simulink model "SC617_Final"  (R2025a)
settings: Solver=ode15s  StartTime=0.0  StopTime=30  MaxStep=0.05  RelTol=1e-2  AbsTol=1e-2
undefined symbols (not defined in the file): magnitude
settings Model: Creator=aayushshah  LastModifiedBy=aayushshah

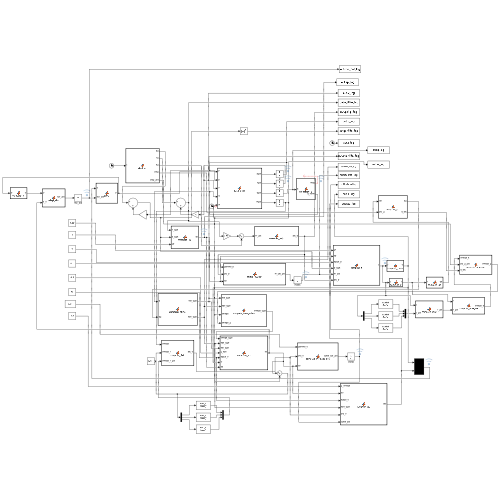
[thumbnail: Simulink's stored preview of the top-level diagram]
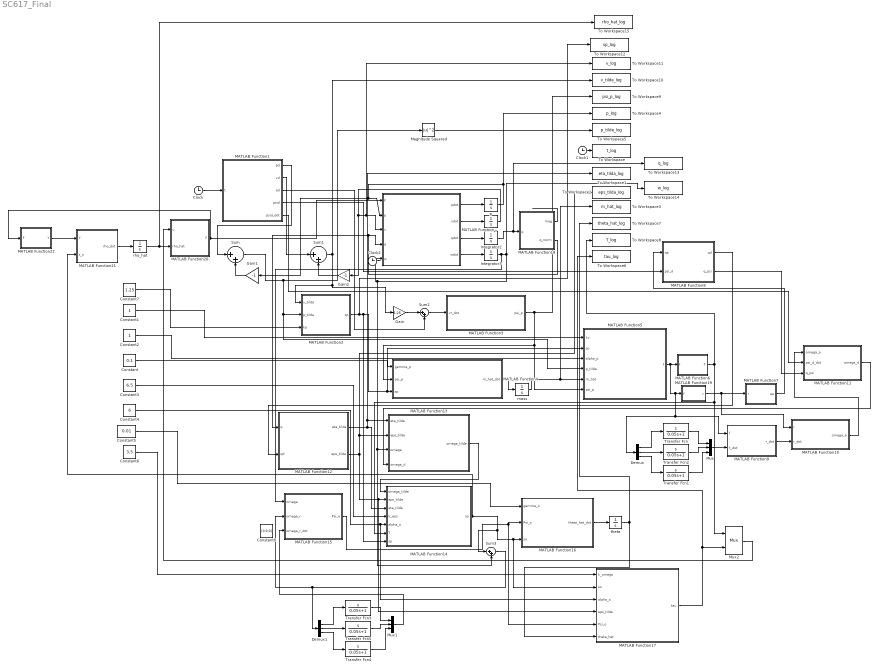
== system SC617_Final ==
  Clock : Clock
  Clock1 : Clock
  Clock2 : Clock
  Constant : Constant  Value=0.1
  Constant1 : Constant
  Constant2 : Constant
  Constant3 : Constant  Value=6.5
  Constant4 : Constant  Value=6
  Constant5 : Constant  Value=0.01
  Constant6 : Constant  Value=3.5
  Constant7 : Constant  Value=1.25
  Constant8 : Constant  Value=[0;0;0]
  Demux : Demux  Outputs=3
  Demux1 : Demux  Outputs=3
  Gain : Gain  Gain=1.25
  Gain1 : Gain  Gain=-1
  Gain2 : Gain  Gain=-1
  Integrator2 : Integrator  InitialCondition=[1; 0; 0; 0]
  Integrator3 : Integrator  InitialCondition=[0; 0; 0]
  MATLAB Function : MATLAB Function  TreatAsAtomicUnit=on
  MATLAB Function1 : MATLAB Function  TreatAsAtomicUnit=on
  MATLAB Function10 : MATLAB Function  TreatAsAtomicUnit=on
  MATLAB Function11 : MATLAB Function  TreatAsAtomicUnit=on
  MATLAB Function12 : MATLAB Function  TreatAsAtomicUnit=on
  MATLAB Function13 : MATLAB Function  TreatAsAtomicUnit=on
  MATLAB Function14 : MATLAB Function  TreatAsAtomicUnit=on
  MATLAB Function15 : MATLAB Function  TreatAsAtomicUnit=on
  MATLAB Function16 : MATLAB Function  TreatAsAtomicUnit=on
  MATLAB Function17 : MATLAB Function  TreatAsAtomicUnit=on
  MATLAB Function18 : MATLAB Function  TreatAsAtomicUnit=on
  MATLAB Function19 : MATLAB Function  TreatAsAtomicUnit=on
  MATLAB Function2 : MATLAB Function  TreatAsAtomicUnit=on
  MATLAB Function20 : MATLAB Function  TreatAsAtomicUnit=on
  MATLAB Function21 : MATLAB Function  TreatAsAtomicUnit=on
  MATLAB Function22 : MATLAB Function  TreatAsAtomicUnit=on
  MATLAB Function3 : MATLAB Function  TreatAsAtomicUnit=on
  MATLAB Function4 : MATLAB Function  TreatAsAtomicUnit=on
  MATLAB Function5 : MATLAB Function  TreatAsAtomicUnit=on
  MATLAB Function6 : MATLAB Function  TreatAsAtomicUnit=on
  MATLAB Function7 : MATLAB Function  TreatAsAtomicUnit=on
  MATLAB Function8 : MATLAB Function  TreatAsAtomicUnit=on
  MATLAB Function9 : MATLAB Function  TreatAsAtomicUnit=on
  Magnitude Squared : Math  Operator=magnitude^2
  Mux : Mux  Inputs=3
  Mux1 : Mux  Inputs=3
  Mux2 : Mux  Inputs=2
  Sum{,1..3} (4 alike) : Sum  Inputs=|++
  To Workspace : ToWorkspace  VariableName=t_log  SampleTime=-1
      settings: Decimation=50  Save2DSignal=2-D array (concatenate along first dimension)
  To Workspace1 : ToWorkspace  VariableName=eta_tilda_log  SampleTime=-1
      settings: Decimation=50  Save2DSignal=2-D array (concatenate along first dimension)
  To Workspace10 : ToWorkspace  VariableName=v_tilde_log  SampleTime=-1
      settings: Decimation=50  Save2DSignal=2-D array (concatenate along first dimension)
  To Workspace11 : ToWorkspace  VariableName=v_log  SampleTime=-1
      settings: Decimation=50  Save2DSignal=2-D array (concatenate along first dimension)
  To Workspace12 : ToWorkspace  VariableName=sp_log  SampleTime=-1
  To Workspace13 : ToWorkspace  VariableName=q_log  SampleTime=-1
      settings: Decimation=50  Save2DSignal=2-D array (concatenate along first dimension)
  To Workspace14 : ToWorkspace  VariableName=w_log  SampleTime=-1
      settings: Decimation=50  Save2DSignal=2-D array (concatenate along first dimension)
  To Workspace15 : ToWorkspace  VariableName=rho_hat_log  SampleTime=-1
  To Workspace2 : ToWorkspace  VariableName=eps_tilda_log  SampleTime=-1
      settings: Decimation=50  Save2DSignal=2-D array (concatenate along first dimension)
  To Workspace3 : ToWorkspace  VariableName=m_hat_log  SampleTime=-1
      settings: Decimation=50  Save2DSignal=2-D array (concatenate along first dimension)
  To Workspace4 : ToWorkspace  VariableName=p_log  SampleTime=-1
      settings: Decimation=50  Save2DSignal=2-D array (concatenate along first dimension)
  To Workspace5 : ToWorkspace  VariableName=p_tilde_log  SampleTime=-1
      settings: Decimation=50  Save2DSignal=2-D array (concatenate along first dimension)
  To Workspace6 : ToWorkspace  VariableName=tau_log  SampleTime=-1
      settings: Decimation=50  Save2DSignal=2-D array (concatenate along first dimension)
  To Workspace7 : ToWorkspace  VariableName=theta_hat_log  SampleTime=-1
      settings: Decimation=50  Save2DSignal=2-D array (concatenate along first dimension)
  To Workspace8 : ToWorkspace  VariableName=T_log  SampleTime=-1
      settings: Decimation=50  Save2DSignal=2-D array (concatenate along first dimension)
  To Workspace9 : ToWorkspace  VariableName=psi_p_log  SampleTime=-1
      settings: Decimation=50  Save2DSignal=2-D array (concatenate along first dimension)
  Transfer Fcn{,1..5} (6 alike) : TransferFcn  Numerator=[1 0]  Denominator=[0.05 1]
  mass : Integrator  InitialCondition=0.8
  p : Integrator  InitialCondition=[4.0; 0.5; 1.0]
  rho_hat : Integrator  InitialCondition=[0.18; 0.009]
  theta : Integrator  InitialCondition=[0.05; 0.05; 0.01]
  v : Integrator  InitialCondition=[0; 0; 0]
  wires:
  MATLAB Function/1(pdot) -> p/1
  MATLAB Function/2(vdot) -> v/1
  MATLAB Function/3(qdot) -> Integrator2/1
  MATLAB Function/4(wdot) -> Integrator3/1
  p/1 -> To Workspace4/1, MATLAB Function/2(p), Gain1/1
  v/1 -> Gain2/1, To Workspace11/1, MATLAB Function/3(v)
  Integrator3/1 -> MATLAB Function15/1(omega), To Workspace14/1, MATLAB Function13/3(omega), Sum3/2, MATLAB Function/5(w)
  Integrator2/1 -> To Workspace13/1, MATLAB Function18/1(q)
  MATLAB Function18/2(q_norm) -> MATLAB Function/4(q), MATLAB Function12/1(q)
  Clock/1 -> MATLAB Function1/1(t)
  MATLAB Function1/1(pd) -> Sum/1
  MATLAB Function1/2(vd) -> Sum1/1
  Sum/1 -> Magnitude Squared/1, MATLAB Function5/4(p_tilda), MATLAB Function2/2(p_tilda)
  Sum1/1 -> MATLAB Function2/1(v_tilda), Gain/1, To Workspace10/1
  Gain/1 -> Sum2/1
  MATLAB Function1/3(ad) -> Sum2/2
  Sum2/1 -> MATLAB Function3/1(vr_dot)
  MATLAB Function2/1(sp) -> To Workspace12/1, MATLAB Function14/7(sp), MATLAB Function5/2(sp), MATLAB Function4/3(sp)
  MATLAB Function3/1(psi_p) -> To Workspace9/1, MATLAB Function5/6(psi_p), MATLAB Function4/2(psi_p)
  Constant/1 -> MATLAB Function4/1(gamma_p)
  Constant1/1 -> MATLAB Function5/1(kv)
  Constant2/1 -> MATLAB Function5/3(alpha_p)
  MATLAB Function5/1(f) -> Demux/1, MATLAB Function9/1(f), MATLAB Function19/1(f), MATLAB Function6/1(f)
  MATLAB Function19/1(r) -> MATLAB Function10/1(r), MATLAB Function7/1(r)
  MATLAB Function7/1(qa) -> MATLAB Function8/1(qa)
  MATLAB Function1/4(psid) -> MATLAB Function8/2(psi_d)
  Demux/1 -> Transfer Fcn/1
  Demux/2 -> Transfer Fcn2/1
  Demux/3 -> Transfer Fcn1/1
  Transfer Fcn/1 -> Mux/1
  Transfer Fcn2/1 -> Mux/2
  Transfer Fcn1/1 -> Mux/3
  MATLAB Function9/1(r_dot) -> MATLAB Function10/2(r_dot)
  MATLAB Function10/1(omega_a) -> MATLAB Function11/1(omega_a)
  MATLAB Function8/2(q_psi) -> MATLAB Function11/3(q_psi)
  MATLAB Function1/5(psid_dot) -> MATLAB Function11/2(psi_d_dot)
  MATLAB Function8/1(qd) -> MATLAB Function12/2(qd)
  MATLAB Function12/1(eta_tilda) -> To Workspace1/1, MATLAB Function13/1(eta_tilde), MATLAB Function14/3(eta_tilde)
  MATLAB Function12/2(eps_tilda) -> MATLAB Function13/2(eps_tilde), To Workspace2/1, MATLAB Function14/2(eps_tilde), MATLAB Function17/4(eps_tilde)
  MATLAB Function11/1(omega_d) -> MATLAB Function13/4(omega_d)
  MATLAB Function13/1(omega_tilde) -> MATLAB Function14/1(omega_tilde)
  MATLAB Function6/1(T) -> To Workspace8/1, Mux2/1, MATLAB Function14/6(T)
  Constant3/1 -> MATLAB Function14/4(k_eps)
  Constant4/1 -> MATLAB Function17/3(alpha_o), MATLAB Function14/5(alpha_o)
  MATLAB Function14/1(so) -> MATLAB Function21/2(s_o), MATLAB Function16/3(so), MATLAB Function17/2(so), Sum3/1
  MATLAB Function15/1(Psi_o) -> MATLAB Function17/5(Psi_o), MATLAB Function16/2(Psi_o)
  Constant5/1 -> MATLAB Function16/1(gamma_o)
  Sum3/1 -> Demux1/1, MATLAB Function15/2(omega_r)
  Transfer Fcn3/1 -> Mux1/1
  Mux1/1 -> MATLAB Function15/3(omega_r_dot)
  Demux1/3 -> Transfer Fcn4/1
  Demux1/2 -> Transfer Fcn5/1
  Demux1/1 -> Transfer Fcn3/1
  Transfer Fcn5/1 -> Mux1/2
  Transfer Fcn4/1 -> Mux1/3
  theta/1 -> MATLAB Function17/6(theta_hat), To Workspace7/1
  Constant6/1 -> MATLAB Function17/1(k_omega)
  MATLAB Function17/1(tau) -> To Workspace6/1, Mux2/2
  Constant7/1 -> MATLAB Function2/3(kp)
  Clock1/1 -> To Workspace/1
  mass/1 -> To Workspace3/1, MATLAB Function5/5(m_hat)
  MATLAB Function16/1(theta_hat_dot) -> theta/1
  MATLAB Function4/1(m_hat_dot) -> mass/1
  Mux2/1 -> MATLAB Function20/1(u)
  Magnitude Squared/1 -> To Workspace5/1
  Mux/1 -> MATLAB Function9/2(f_dot)
  MATLAB Function18/1(mag) -> ?
  Gain1/1 -> Sum/2
  Gain2/1 -> Sum1/2
  Clock2/1 -> ?
  MATLAB Function20/1(F) -> MATLAB Function22/1(F), MATLAB Function/1(F)
  MATLAB Function21/1(rho_dot) -> rho_hat/1
  rho_hat/1 -> To Workspace15/1, MATLAB Function20/2(rho_hat)
  MATLAB Function22/1(Y) -> MATLAB Function21/1(Y)

== matlab function SC617_Final/MATLAB Function9 ==
  data: f input; r_dot output; f_dot input
function r_dot = compute_rdot(f, f_dot)
    nf = norm(f);
    if nf < 0.1
        r_dot = [0; 0; 0];
    else
        r_dot = (1/nf)*(eye(3) - (f*f')/(nf^2))*f_dot;
    end
end

== matlab function SC617_Final/MATLAB Function10 ==
  data: r input; omega_a output; r_dot input
function omega_a = compute_omegaa(r, r_dot)
    rx = r(1);   ry = r(2);   rz = r(3);
    rxd = r_dot(1); ryd = r_dot(2); rzd = r_dot(3);
    
    denom = 1 + rz;
    
    if abs(denom) < 1e-6
        omega_a = [0; 0; 0];
        return;
    end
    
    omega_a = [ (-ryd*denom + ry*rzd) / denom;
                ( rxd*denom - rx*rzd) / denom;
                ( ry*rxd - rx*ryd)    / denom ];
end

== matlab function SC617_Final/MATLAB Function11 ==
  data: omega_a input; omega_d output; psi_d_dot input; q_psi input
function omega_d = compute_omegad(omega_a, psi_d_dot, q_psi)
    omega_psi = [0; 0; psi_d_dot];
    q_inv = [q_psi(1); -q_psi(2); -q_psi(3); -q_psi(4)];
    eta = q_inv(1);
    eps = q_inv(2:4);
    omega_a_rot = (eta^2 - eps'*eps)*omega_a ...
                + 2*(eps'*omega_a)*eps ...
                + 2*eta*cross(eps, omega_a);
    omega_d = omega_psi + omega_a_rot;
end

== matlab function SC617_Final/MATLAB Function12 ==
  data: q input; eta_tilda output; qd input; eps_tilda output
function [eta_tilda, eps_tilda] = compute_qtilde(q, qd)
    eta = q(1);
    eps = q(2:4);
    eta_d = qd(1);
    eps_d = qd(2:4);
    eta_inv = eta;
    eps_inv = -eps;  
    eta_tilda = eta_inv*eta_d - dot(eps_inv,eps_d);
    eps_tilda = eta_inv.*eps_d + eta_d.*eps_inv + cross(eps_inv, eps_d);
end

== matlab function SC617_Final/MATLAB Function13 ==
  data: eta_tilde input; omega_tilde output; eps_tilde input; omega input; omega_d input
function omega_tilde = compute_omegatilde(eta_tilde, eps_tilde, omega, omega_d)
    eta = eta_tilde; eps = eps_tilde;
    omega_d_rot = (eta^2 - dot(eps,eps))*omega_d ...
                + 2*(dot(eps,omega_d))*eps ...
                + 2*eta*cross(eps, omega_d);
    
    omega_tilde = omega_d_rot - omega;
end

== matlab function SC617_Final/MATLAB Function14 ==
  data: omega_tilde input; eps_tilde input; eta_tilde input; so output; k_eps input; alpha_o input; T input; sp input
function so = compute_so(omega_tilde, eps_tilde, eta_tilde, ...
                          k_eps, alpha_o, T, sp)
   
   
    eps_bar = [eps_tilde(2); -eps_tilde(1); eta_tilde];
    
    % S(eps_bar) skew matrix
    S_epsbar = [    0       -eps_bar(3)  eps_bar(2);
               eps_bar(3)      0        -eps_bar(1);
              -eps_bar(2)  eps_bar(1)       0      ];
    eta = eta_tilde;
    eps = -eps_tilde;
    
    sp_rot = (eta^2 - eps'*eps)*sp ...
           + 2*(eps'*sp)*eps ...
           + 2*eta*cross(eps, sp);
    so = omega_tilde + k_eps*eps_tilde + 2*(1/alpha_o)*T*S_epsbar*sp_rot;
end

== matlab function SC617_Final/MATLAB Function1 ==
  data: t input; pd output; vd output; ad output; psid output; psid_dot output
function [pd, vd, ad, psid, psid_dot] = desired(t)

pd = [2*cos(0.4*t) + 0.5*sin(1.0*t);2*sin(0.4*t) + 0.5*cos(1.2*t); 2 + 0.4*sin(0.6*t)];

vd = [-2*0.4*sin(0.4*t) + 0.5*1.0*cos(1.0*t); ...
     2*0.4*cos(0.4*t) - 0.5*1.2*sin(1.2*t); ...
     0.4*0.6*cos(0.6*t) ...
];

ad = [ -2*(0.4)^2*cos(0.4*t) - 0.5*(1.0)^2*sin(1.0*t); ...
    -2*(0.4)^2*sin(0.4*t) - 0.5*(1.2)^2*cos(1.2*t); ...
    -0.4*(0.6)^2*sin(0.6*t) ...
];

psid = (pi/6)*sin(0.5*t);
psid_dot = (pi/6)*0.5*cos(0.5*t);

end

== matlab function SC617_Final/MATLAB Function15 ==
  data: omega input; Psi_o output; omega_r input; omega_r_dot input
function Psi_o = compute_Psio(omega, omega_r, omega_r_dot)
    S_omegar = [  0          -omega_r(3)   omega_r(2);
               omega_r(3)    0            -omega_r(1);
              -omega_r(2)    omega_r(1)    0          ];
    Psi_o = [omega_r_dot(1)   S_omegar(1,2)*omega(2)   S_omegar(1,3)*omega(3);
             S_omegar(2,1)*omega(1)   omega_r_dot(2)   S_omegar(2,3)*omega(3);
             S_omegar(3,1)*omega(1)   S_omegar(3,2)*omega(2)   omega_r_dot(3)];
end

== matlab function SC617_Final/MATLAB Function16 ==
  data: gamma_o input; theta_hat_dot output; Psi_o input; so input
function theta_hat_dot = compute_thetahat_dot(gamma_o, Psi_o, so)
    theta_hat_dot = gamma_o * (Psi_o' * so);
end

== matlab function SC617_Final/MATLAB Function17 ==
  data: k_omega input; tau output; so input; alpha_o input; eps_tilde input; Psi_o input; theta_hat input
function tau = compute_tau(k_omega, so, alpha_o, eps_tilde, Psi_o, theta_hat)
    tau = k_omega*so + alpha_o*eps_tilde + Psi_o*theta_hat;
end

== matlab function SC617_Final/MATLAB Function18 ==
  data: mag output; q input; q_norm output
function [mag, q_norm] = normalize_q(q)
    q_norm = q / norm(q);
    mag = norm(q_norm);
end

== matlab function SC617_Final/MATLAB Function19 ==
  data: f input; r output
function r = compute_r(f)
    nf = norm(f);
    if nf < 0.1      
        r = [0; 0; 1];
    else
        r = f / nf;
    end
end

== matlab function SC617_Final/MATLAB Function20 ==
  data: u input; F output; rho_hat input
function F = alloc(u, rho_hat)
f  = u(1);
Mx = u(2);
My = u(3);
Mz = u(4);
l  = rho_hat(1);
kM = rho_hat(2);
A = [
    1  1  1  1;
   -sqrt(2)/2*l   sqrt(2)/2*l   sqrt(2)/2*l  -sqrt(2)/2*l;
    sqrt(2)/2*l  -sqrt(2)/2*l   sqrt(2)/2*l  -sqrt(2)/2*l;
    kM  kM  -kM  -kM];
F = A \ [f; Mx; My; Mz];
F = max(F, 0);
end

== matlab function SC617_Final/MATLAB Function21 ==
  data: Y input; rho_dot output; s_o input
function rho_dot = adapt_rho(Y, s_o)

gamma = diag([0.0005, 0.0005]);

rho_dot = -gamma * Y' * s_o;
rho_dot = max(min(rho_dot, 0.05), -0.05);

end

== matlab function SC617_Final/MATLAB Function22 ==
  data: F input; Y output
function Y = compute_Y(F)

F1 = F(1);
F2 = F(2);
F3 = F(3);
F4 = F(4);

phi_x = (sqrt(2)/2)*(-F1 + F2 + F3 - F4);
phi_y = (sqrt(2)/2)*( F1 - F2 + F3 - F4);
phi_z = (F1 + F2 - F3 - F4);

Y = [phi_x, 0;
     phi_y, 0;
     0,     phi_z];
end

== matlab function SC617_Final/MATLAB Function ==
  data: F input; p input; v input; q input; w input; pdot output; vdot output; qdot output; wdot output
function [pdot, vdot, qdot, wdot] = quad_plant(F, p, v, q, w)
m = 1.0;
g = 9.81;
J = diag([0.01, 0.01, 0.02]);

l  = 0.2;      
c2 = 1.0;    
c1 = 0.01;    

kM = c1 / c2;

e3 = [0;0;1];


F1 = F(1);
F2 = F(2);
F3 = F(3);
F4 = F(4);

f = F1 + F2 + F3 + F4;

Mx = (-sqrt(2)/2*l)*F1 + ( sqrt(2)/2*l)*F2 + ( sqrt(2)/2*l)*F3 + (-sqrt(2)/2*l)*F4;

My = ( sqrt(2)/2*l)*F1 + (-sqrt(2)/2*l)*F2 + ( sqrt(2)/2*l)*F3 + (-sqrt(2)/2*l)*F4;

Mz = kM*F1 + kM*F2 - kM*F3 - kM*F4;

tau = [Mx; My; Mz];


eta = q(1);
eps = q(2:4);

R = (eta^2 - eps'*eps)*eye(3) + 2*(eps*eps') + 2*eta*skew(eps);


pdot = v;
vdot = (f/m)*R*e3 - g*e3;


wdot = J \ (tau - cross(w, J*w));
Omega = [    0, -w(1), -w(2), -w(3);
          w(1),     0, -w(3),  w(2);
          w(2),  w(3),     0, -w(1);
          w(3), -w(2),  w(1),     0];

qdot = 0.5 * Omega * q;
qdot = qdot - (q' * qdot) * q;

end

function S = skew(v)
S = [  0   -v(3)  v(2);
     v(3)   0   -v(1);
    -v(2)  v(1)   0 ];
end

== matlab function SC617_Final/MATLAB Function2 ==
  data: v_tilda input; sp output; p_tilda input; kp input
function sp = compute_sp(v_tilda, p_tilda, kp)
    sp = v_tilda + kp*p_tilda;
end

== matlab function SC617_Final/MATLAB Function3 ==
  data: vr_dot input; psi_p output
function psi_p = compute_psip(vr_dot)
    g = 9.81;
    zi = [0; 0; 1];
    psi_p = vr_dot + g*zi;
end

== matlab function SC617_Final/MATLAB Function4 ==
  data: gamma_p input; m_hat_dot output; psi_p input; sp input
function m_hat_dot = mass_update(gamma_p, psi_p, sp)
    m_hat_dot = gamma_p * (psi_p' * sp);
end

== matlab function SC617_Final/MATLAB Function5 ==
  data: kv input; f output; sp input; alpha_p input; p_tilda input; m_hat input; psi_p input
function f = compute_f(kv, sp, alpha_p, p_tilda, m_hat, psi_p)
    f = kv*sp + alpha_p*p_tilda+ m_hat*psi_p;
end

== matlab function SC617_Final/MATLAB Function6 ==
  data: f input; T output
function T = compute_thrust(f)
    T = norm(f);
end

== matlab function SC617_Final/MATLAB Function7 ==
  data: r input; qa output
function qa = compute_qa(r)
    if r(3) < -0.999999
        qa = [0; 1; 0; 0];
        return;
    end
    qa_raw = [1 + r(3);
             -r(2);
              r(1);
              0];
    qa = qa_raw / norm(qa_raw);
end

== matlab function SC617_Final/MATLAB Function8 ==
  data: qa input; qd output; psi_d input; q_psi output
function [qd, q_psi] = compute_qd(qa, psi_d)
    q_psi = [cos(psi_d/2); 0; 0; sin(psi_d/2)];
    qd = quat_multiply(qa, q_psi);
end

function q = quat_multiply(q1, q2)
    eta1 = q1(1); eps1 = q1(2:4);
    eta2 = q2(1); eps2 = q2(2:4);
    eta = eta1*eta2 - eps1'*eps2;
    eps = eta1*eps2 + eta2*eps1 + cross(eps1, eps2);
    q = [eta; eps];
end
